simulink model "Generate_Duty_Cycle"  (R2025a)
settings: Solver=ode23tb  StartTime=0.0  StopTime=0.001  MaxStep=1e-4  RelTol=1e-3
libraries: simulink x1, spspowerguiLib x1
settings Model: Creator=Jawad  LastModifiedBy=Jawad

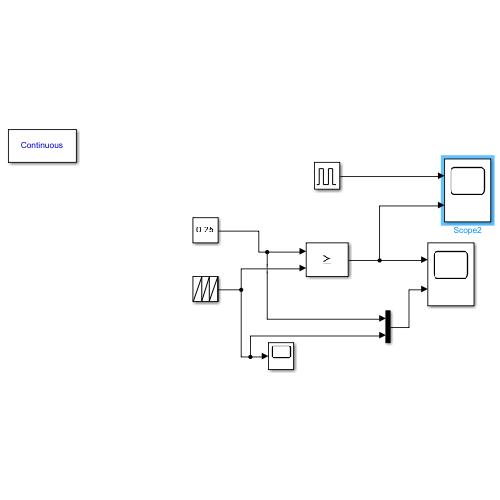
[thumbnail: Simulink's stored preview of the top-level diagram]
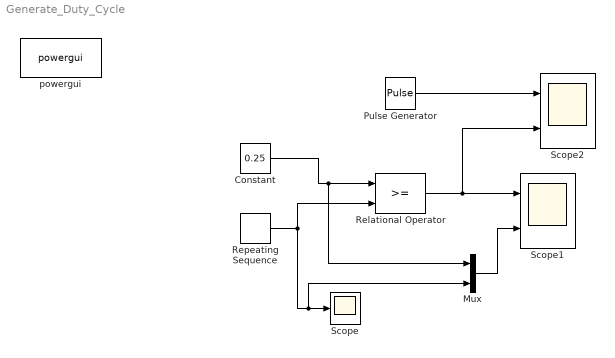
== system Generate_Duty_Cycle ==
  Constant : Constant  Value=0.25
  Mux : Mux  Inputs=2
  Pulse Generator : DiscretePulseGenerator  PulseType=Time based  Period=1/5000  PulseWidth=25
  Relational Operator : RelationalOperator  OutDataTypeStr=boolean  RndMeth=Simplest  InputSameDT=off
  Repeating Sequence : simulink/Sources/Repeating Sequence  rep_seq_t=[0 1/5000]  rep_seq_y=[0 1]
  Scope : Scope
      settings: ActiveDisplayYMinimum=-0.26580543730625927  ActiveDisplayYMaximum=1.3517764310467919
  Scope1 : Scope  NumInputPorts=2
      settings: ActiveDisplayYMinimum=0.8716624063261702  ActiveDisplayYMaximum=1.1897533163861105
  Scope2 : Scope  NumInputPorts=2
      settings: ActiveDisplayYMinimum=-0.12499999999999997  ActiveDisplayYMaximum=1.125  DataLoggingVariableName=ScopeData2
  powergui : spspowerguiLib/powergui  Priority=1  SimulationMode=Continuous  SampleTime=50e-6  frequency=60  Iterations=50  frequencyindice=60  Pbase=100e6  ErrMax=1e-4  UnitsV=kV  UnitsW=MW  buscounter=0  FunctionMessages=off  echomessages=off  EnableUseOfTLC=off  CurrentSourceSwitches=off  DisableSnubberDevices=off  DisableRonSwitches=off  DisableVfSwitches=off  DisplayEquations=off  AutomaticDiscreteSolvers=off  SolverType=Tustin/Backward Euler (TBE)  Interpol=off  ExternalGateDelay=off  methode=off  Ts=100  x0status=blocks  SPID=on  SwTol=0  HookPort=off  NonlinearTolerance=1e-4  nMaxIteration=100  ContinueOnMaxIteration=off  RestoreLinks=warning  ResistiveCurrentMeasurement=off  Frange=[0:2:500]  Ylog=off  Xlog=on  ShowGrid=off  save=off  variable=ZData  structure=0  ZoomFFT=off  StartTime=0.0  cycles=1  DisplayStyle=1  fundamental=60  FreqAxis=off  MaxFrequency=1000  frequencyindicesteady=1  RmsSteady=1  display=off
  wires:
  Constant/1 -> Mux/1, Relational Operator/1
  Repeating Sequence/1 -> Mux/2, Scope/1, Relational Operator/2
  Relational Operator/1 -> Scope2/2, Scope1/1
  Mux/1 -> Scope1/2
  Pulse Generator/1 -> Scope2/1
